simulink model "EcoSIM3_P2_C2_WIP"  (R2014b)
settings: Solver=ode1  SolverMode=SingleTasking  StartTime=0.0  StopTime=4  FixedStep=0.01  RelTol=1e-3
PostLoadFcn:
  | %, if any(exist('dsrtsu_mdlpostloadfcn', 'file') == [2, 3, 6]), try dsrtsu_mdlpostloadfcn('Execute', bdroot); catch fprintf('Error in PostLoadFcn (dsrtsu_mdlpostloadfcn) for model "%s":\n %s\n', bdroot, lasterr); end, end,
InitFcn:
  | tic
  | %Startup_EcoSIM
undefined symbols (not defined in the file or in its folder): canChannel, Controls, DriveCycles, Driver, EM_EFF_MAP, EM_PwrLoss_MAP, EngPwr, EngSpd, EngTrq, Glbl, Overwritten_Mode, Plants, Power, sigbuilder_block, Torque, Trialmap, Veh_Dynamics
libraries: simulink x135, canmsglib x113, fl_lib x104, canlib x89, nesl_utility x56, sdl_lib x29, dspsigops x6, dspswit3 x5, dspstat3 x2, commnoisgen2 x1, dspfdesign x1
(part 14 of 21)

== system EcoSIM3_P2_C2_WIP/Supervisory Controller/Supervisory_IO/VNT Kvaser/CAN Tx/ICE_BAS_Trans ==
  ICE_BAS_Trans : Inport
  Bus Selector1 : BusSelector  OutputSignals=ICE_Torque_Request_Nm,BAS_SoftECU_Receive.BAS_Mode_Request,BAS_SoftECU_Receive.BAS_Torque_Request_Nm,Trans_Receive.Gear_Request
  CAN Pack1 : canmsglib/CAN Pack  CANdbFile=C:\Users\EcoCAR_HIL\Documents\Khanna\EcoSIM3_P1_0_PHEV_TCU\Final_DBC\Engine_Transmission_BAS.dbc  MsgList=ECO_Engine_MSG101  MsgName=ECO_Engine_MSG101  MsgIDType=Standard (11-bit identifier)  MsgIdentifier=101  MsgLength=2  SignalInfo=ICE_Torque_Request_Nm$9$15$2$2$1$0$1.000000e-02$0$0$3.276700e+02$#  NSignals=1  StartBits=str2num('[int32(9)]')  SignalSizes=str2num('[int32(15)]')  ByteOrders=str2num('[int32(2)]')  DataTypes=str2num('[int32(2)]')  MultiplexTypes=str2num('[int32(1)]')  MultiplexValues=str2num('[double(0)]')  Factors=str2num('[double(1.000000e-02)]')  Offsets=str2num('[double(0)]')  Minimums=str2num('[double(0)]')  Maximums=str2num('[double(3.276700e+02)]')  Remote=off
      settings: DataFormat=CANdb specified signals
  CAN Pack2 : canmsglib/CAN Pack  CANdbFile=C:\Users\EcoCAR_HIL\Documents\Khanna\EcoSIM3_P1_0_PHEV_TCU\Final_DBC\Engine_Transmission_BAS.dbc  MsgList=ECO_BAS_Receive_MSG102  MsgName=ECO_BAS_Receive_MSG102  MsgIDType=Standard (11-bit identifier)  MsgIdentifier=102  MsgLength=2  SignalInfo=BAS_Mode_Request$8$1$2$2$1$0$1$0$0$1$#BAS_Torque_Request_Nm$9$15$2$1$1$0$1.000000e-02$0$-1.638400e+02$1.638300e+02$#  NSignals=2  StartBits=str2num('[int32(8);int32(9)]')  SignalSizes=str2num('[int32(1);int32(15)]')  ByteOrders=str2num('[int32(2);int32(2)]')  DataTypes=str2num('[int32(2);int32(1)]')  MultiplexTypes=str2num('[int32(1);int32(1)]')  MultiplexValues=str2num('[double(0);double(0)]')  Factors=str2num('[double(1);double(1.000000e-02)]')  Offsets=str2num('[double(0);double(0)]')  Minimums=str2num('[double(0);double(-1.638400e+02)]')  Maximums=str2num('[double(1);double(1.638300e+02)]')  Remote=off
      settings: DataFormat=CANdb specified signals
  CAN Pack3 : canmsglib/CAN Pack  CANdbFile=C:\Users\EcoCAR_HIL\Documents\Khanna\EcoSIM3_P1_0_PHEV_TCU\Final_DBC\Engine_Transmission_BAS.dbc  MsgList=ECO_Trans_Receive_MSG105  MsgName=ECO_Trans_Receive_MSG105  MsgIDType=Standard (11-bit identifier)  MsgIdentifier=105  MsgLength=1  SignalInfo=Clutch_Request$4$1$2$2$1$0$1$0$0$1$#Gear_Request$5$3$2$2$1$0$1$0$0$7$#  NSignals=2  StartBits=str2num('[int32(4);int32(5)]')  SignalSizes=str2num('[int32(1);int32(3)]')  ByteOrders=str2num('[int32(2);int32(2)]')  DataTypes=str2num('[int32(2);int32(2)]')  MultiplexTypes=str2num('[int32(1);int32(1)]')  MultiplexValues=str2num('[double(0);double(0)]')  Factors=str2num('[double(1);double(1)]')  Offsets=str2num('[double(0);double(0)]')  Minimums=str2num('[double(0);double(0)]')  Maximums=str2num('[double(1);double(7)]')  Remote=off
      settings: DataFormat=CANdb specified signals
  CAN Transmit1 : canlib/CAN Transmit  BlockHandle=7844.0023  DeviceMenu=Kvaser Virtual 1 (Channel 1)  Device=Kvaser Virtual 1 (Channel 1)  ObjConstructor=canChannel('Kvaser', 'Virtual 1', 1)  EnablePeriodicTransmit=off  MessagePeriod=1.000
  CAN Transmit2 : canlib/CAN Transmit  BlockHandle=7845.0023  DeviceMenu=Kvaser Virtual 1 (Channel 1)  Device=Kvaser Virtual 1 (Channel 1)  ObjConstructor=canChannel('Kvaser', 'Virtual 1', 1)  EnablePeriodicTransmit=off  MessagePeriod=1.000
  CAN Transmit3 : canlib/CAN Transmit  BlockHandle=7846.0023  DeviceMenu=Kvaser Virtual 1 (Channel 1)  Device=Kvaser Virtual 1 (Channel 1)  ObjConstructor=canChannel('Kvaser', 'Virtual 1', 1)  EnablePeriodicTransmit=off  MessagePeriod=1.000
  Ground1 : Ground
  Rate Transition{,1..3} (4 alike) : RateTransition
  wires:
  ICE_BAS_Trans/1 -> Bus Selector1/1
  Ground1/1 -> CAN Pack3/1
  CAN Pack2/1 -> CAN Transmit2/1
  Bus Selector1/3 -> Rate Transition2/1  "<BAS_Torque_Request_Nm>"
  Bus Selector1/2 -> Rate Transition1/1  "<BAS_Mode_Request>"
  CAN Pack3/1 -> CAN Transmit3/1
  Bus Selector1/4 -> Rate Transition3/1  "<Gear_Request>"
  CAN Pack1/1 -> CAN Transmit1/1
  Bus Selector1/1 -> Rate Transition/1  "<ICE_Torque_Request_Nm>"
  Rate Transition/1 -> CAN Pack1/1
  Rate Transition1/1 -> CAN Pack2/1
  Rate Transition2/1 -> CAN Pack2/2
  Rate Transition3/1 -> CAN Pack3/2

== system EcoSIM3_P2_C2_WIP/Supervisory Controller/Supervisory_IO/VNT Kvaser/CAN Tx/Mode ==
  Mode : Inport
  Bus Selector3 : BusSelector  OutputSignals=Supervisory.Mode
  CAN Pack5 : canmsglib/CAN Pack  CANdbFile=C:\Users\EcoCAR_HIL\Documents\Khanna\EcoSIM3_P1_0_PHEV_TCU\Final_DBC\EcoCAR3_Controls_Development.dbc  MsgList=MABx_Transmit_MSG094  MsgName=MABx_Transmit_MSG094  MsgIDType=Standard (11-bit identifier)  MsgIdentifier=94  MsgLength=1  SignalInfo=Mode$7$1$2$2$1$0$1$0$0$1$#  NSignals=1  StartBits=str2num('[int32(7)]')  SignalSizes=str2num('[int32(1)]')  ByteOrders=str2num('[int32(2)]')  DataTypes=str2num('[int32(2)]')  MultiplexTypes=str2num('[int32(1)]')  MultiplexValues=str2num('[double(0)]')  Factors=str2num('[double(1)]')  Offsets=str2num('[double(0)]')  Minimums=str2num('[double(0)]')  Maximums=str2num('[double(1)]')  Remote=off
      settings: DataFormat=CANdb specified signals
  CAN Transmit5 : canlib/CAN Transmit  BlockHandle=7869.0023  DeviceMenu=Kvaser Virtual 1 (Channel 1)  Device=Kvaser Virtual 1 (Channel 1)  ObjConstructor=canChannel('Kvaser', 'Virtual 1', 1)  EnablePeriodicTransmit=off  MessagePeriod=1.000
  Data Type Conversion1 : DataTypeConversion
  Rate Transition : RateTransition
  wires:
  Mode/1 -> Bus Selector3/1
  Data Type Conversion1/1 -> Rate Transition/1  "Mode"
  CAN Pack5/1 -> CAN Transmit5/1
  Bus Selector3/1 -> Data Type Conversion1/1  "<Mode>"
  Rate Transition/1 -> CAN Pack5/1

== system EcoSIM3_P2_C2_WIP/Supervisory Controller/Supervisory_IO/VNT Vector/CAN Rx/BAS ==
  Bus Creator : BusCreator  Inputs=2
  Bus Creator1 : BusCreator  Inputs=2
  Bus Creator2 : BusCreator  Inputs=3
  CAN Receive5 : canlib/CAN Receive  BlockHandle=17800.0002  DeviceMenu=Vector Virtual 1 (Channel 1)  Device=Vector Virtual 1 (Channel 1)  ObjConstructor=canChannel('Vector', 'Virtual 1', 1)  EnableStandardIDsFilter=off  StandardIDs=[257 273]  EnableExtendedIDsFilter=off  ExtendedIDs=0  SampleTime=0.01  MsgsPerTimestep=1  StdIDsCombo=Allow only  ExtIDsCombo=Block all  InternalFilterUpdateStatus=on
  CAN Unpack1 : canmsglib/CAN Unpack  CANdbFile=C:\Box Sync\EcoCAR 3\SMS\EcoSIM3_P2_C2\MIL\Final_DBC\InfineonInverter.dbc  MsgList=Status_1  MsgName=Status_1  MsgIDType=Standard (11-bit identifier)  MsgIdentifier=257  MsgLength=8  SignalInfo=Checksum3$0$8$1$2$1$0$1$0$-Inf$Inf$#CoolingReq$55$1$1$2$1$0$1$0$0$1$#Counter3$8$8$1$2$1$0$1$0$0$15$#ErrorInfo$48$2$1$2$1$0$1$0$0$3$#PowerRed$50$4$1$2$1$0$1$0$0$15$#ReadyHV$54$1$1$2$1$0$1$0$0$1$#RegAtLimit$56$1$1$2$1$0$1$0$0$1$#Reserved4$59$1$1$2$1$0$1$0$0$1$#SetLimitsOk$57$1$1$2$1$0$1$0$0$1$#SetValuesOk$58$1$1$2$1$0$1$0$0$1$#Speed$32$16$1$1$1$0$5.000000e-01$0$-16384$1.638350e+04$#StatusMode$60$4$1$2$1$0$1$0$0$15$#Torque_Normalized$16$16$1$1$1$0$3.051758e-05$0$-1$9.999695e-01$#  NSignals=13  IDPort=off  TimestampPort=off  ErrorPort=off  RemotePort=off  LengthPort=off  StatusPort=off  StartBits=str2num('[int32(0);int32(55);int32(8);int32(48);int32(50);int32(54);int32(56);int32(59);int32(57);int32(58);int32(32);int32(60);int32(16)]')  SignalSizes=str2num('[int32(8);int32(1);int32(8);int32(2);int32(4);int32(1);int32(1);int32(1);int32(1);int32(1);int32(16);int32(4);int32(16)]')  ByteOrders=str2num('[int32(1);int32(1);int32(1);int32(1);int32(1);int32(1);int32(1);int32(1);int32(1);int32(1);int32(1);int32(1);int32(1)]')  DataTypes=str2num('[int32(2);int32(2);int32(2);int32(2);int32(2);int32(2);int32(2);int32(2);int32(2);int32(2);int32(1);int32(2);int32(1)]')  MultiplexTypes=str2num('[int32(1);int32(1);int32(1);int32(1);int32(1);int32(1);int32(1);int32(1);int32(1);int32(1);int32(1);int32(1);int32(1)]')  MultiplexValues=str2num('[double(0);double(0);double(0);double(0);double(0);double(0);double(0);double(0);double(0);double(0);double(0);double(0);double(0)]')  Factors=str2num('[double(1);double(1);double(1);double(1);double(1);double(1);double(1);double(1);double(1);double(1);double(5.000000e-01);double(1);double(3.051758e-05)]')  Offsets=str2num('[double(0);double(0);double(0);double(0);double(0);double(0);double(0);double(0);double(0);double(0);double(0);double(0);double(0)]')  Minimums=str2num('[double(-Inf);double(0);double(0);double(0);double(0);double(0);double(0);double(0);double(0);double(0);double(-16384);double(0);double(-1)]')  Maximums=str2num('[double(Inf);double(1);double(15);double(3);double(15);double(1);double(1);double(1);double(1);double(1);double(1.638350e+04);double(15);double(9.999695e-01)]')
      settings: DataFormat=CANdb specified signals
  CAN Unpack2 : canmsglib/CAN Unpack  CANdbFile=C:\Box Sync\EcoCAR 3\SMS\EcoSIM3_P2_C2\MIL\Final_DBC\InfineonInverter.dbc  MsgList=Status_2  MsgName=Status_2  MsgIDType=Standard (11-bit identifier)  MsgIdentifier=273  MsgLength=8  SignalInfo=Checksum4$0$8$1$2$1$0$1$0$-Inf$Inf$#Counter4$8$4$1$2$1$0$1$0$0$15$#CurrentD_Limit$32$16$1$1$3$7$3.125000e-02$0$-1024$1.023969e+03$#CurrentD_Reference$32$16$1$1$3$9$3.125000e-02$0$-1024$1.023969e+03$#CurrentQ_Limit$32$16$1$1$3$6$3.125000e-02$0$-1024$1.023969e+03$#CurrentQ_Reference$32$16$1$1$3$8$3.125000e-02$0$-1024$1.023969e+03$#FaultU$13$1$1$2$1$0$1$0$0$1$#FaultV$14$1$1$2$1$0$1$0$0$1$#FaultW$15$1$1$2$1$0$1$0$0$1$#MultiplexCode$48$16$1$2$2$0$1$0$0$65535$#PhaseU_IGBT_Temp$32$16$1$1$3$3$7.812500e-03$0$-256$2.559922e+02$#PhaseV_IGBT_Temp$32$16$1$1$3$4$7.812500e-03$0$-256$2.559922e+02$#PhaseW_IGBT_Temp$32$16$1$1$3$5$7.812500e-03$0$-256$2.559922e+02$#RehabilitationReq$12$1$1$2$1$0$1$0$0$1$#Software_Version$32$16$1$2$3$0$1$0$0$65535$#Speed_Command$32$16$1$1$3$1$5.000000e-01$0$-16384$1.638350e+04$#Stator_Temperature$32$16$1$1$3$2$7.812500e-03$0$-256$2.559922e+02$#VoltageDC$16$16$1$1$1$0$3.125000e-02$0$-1024$1.023969e+03$#  NSignals=18  IDPort=off  TimestampPort=off  ErrorPort=off  RemotePort=off  LengthPort=off  StatusPort=off  StartBits=str2num('[int32(0);int32(8);int32(32);int32(32);int32(32);int32(32);int32(13);int32(14);int32(15);int32(48);int32(32);int32(32);int32(32);int32(12);int32(32);int32(32);int32(32);int32(16)]')  SignalSizes=str2num('[int32(8);int32(4);int32(16);int32(16);int32(16);int32(16);int32(1);int32(1);int32(1);int32(16);int32(16);int32(16);int32(16);int32(1);int32(16);int32(16);int32(16);int32(16)]')  ByteOrders=str2num('[int32(1);int32(1);int32(1);int32(1);int32(1);int32(1);int32(1);int32(1);int32(1);int32(1);int32(1);int32(1);int32(1);int32(1);int32(1);int32(1);int32(1);int32(1)]')  DataTypes=str2num('[int32(2);int32(2);int32(1);int32(1);int32(1);int32(1);int32(2);int32(2);int32(2);int32(2);int32(1);int32(1);int32(1);int32(2);int32(2);int32(1);int32(1);int32(1)]')  MultiplexTypes=str2num('[int32(1);int32(1);int32(3);int32(3);int32(3);int32(3);int32(1);int32(1);int32(1);int32(2);int32(3);int32(3);int32(3);int32(1);int32(3);int32(3);int32(3);int32(1)]')  MultiplexValues=str2num('[double(0);double(0);double(7);double(9);double(6);double(8);double(0);double(0);double(0);double(0);double(3);double(4);double(5);double(0);double(0);double(1);double(2);double(0)]')  Factors=str2num('[double(1);double(1);double(3.125000e-02);double(3.125000e-02);double(3.125000e-02);double(3.125000e-02);double(1);double(1);double(1);double(1);double(7.812500e-03);double(7.812500e-03);double(7.812500e-03);double(1);double(1);double(5.000000e-01);double(7.812500e-03);double(3.125000e-02)]')  Offsets=str2num('[double(0);double(0);double(0);double(0);double(0);double(0);double(0);double(0);double(0);double(0);double(0);double(0);double(0);double(0);double(0);double(0);double(0);double(0)]')  Minimums=str2num('[double(-Inf);double(0);double(-1024);double(-1024);double(-1024);double(-1024);double(0);double(0);double(0);double(0);double(-256);double(-256);double(-256);double(0);double(0);double(-16384);double(-256);double(-1024)]')  Maximums=str2num('[double(Inf);double(15);double(1.023969e+03);double(1.023969e+03);double(1.023969e+03);double(1.023969e+03);double(1);double(1);double(1);double(65535);double(2.559922e+02);double(2.559922e+02);double(2.559922e+02);double(1);double(65535);double(1.638350e+04);double(2.559922e+02);double(1.023969e+03)]')
      settings: DataFormat=CANdb specified signals
  Terminator2 : Terminator
  Terminator_{2..27} (26 alike) : Terminator
  BAS : Outport
  wires:
  CAN Unpack2/9 -> Bus Creator2/3  "Fault_W"
  CAN Unpack2/8 -> Bus Creator2/2  "Fault_V"
  CAN Unpack2/7 -> Bus Creator2/1  "Fault_U"
  CAN Unpack1/13 -> Bus Creator1/2  "BAS_Torque_Out_Nm"
  CAN Unpack1/11 -> Bus Creator1/1  "BAS_Speed_rad_per_s"
  Bus Creator1/1 -> Bus Creator/1  "Status_1"
  Bus Creator2/1 -> Bus Creator/2  "Status_2"
  Bus Creator/1 -> BAS/1  "BAS_CAN_Out"
  CAN Receive5/2 -> CAN Unpack1/1, CAN Unpack2/1
  CAN Receive5/1 -> Terminator2/1
  CAN Unpack1/1 -> Terminator_2/1
  CAN Unpack1/2 -> Terminator_3/1
  CAN Unpack1/3 -> Terminator_4/1
  CAN Unpack1/4 -> Terminator_5/1
  CAN Unpack1/5 -> Terminator_6/1
  CAN Unpack1/6 -> Terminator_7/1
  CAN Unpack1/7 -> Terminator_8/1
  CAN Unpack1/8 -> Terminator_9/1
  CAN Unpack1/9 -> Terminator_10/1
  CAN Unpack1/10 -> Terminator_11/1
  CAN Unpack1/12 -> Terminator_12/1
  CAN Unpack2/1 -> Terminator_13/1
  CAN Unpack2/2 -> Terminator_14/1
  CAN Unpack2/3 -> Terminator_15/1
  CAN Unpack2/4 -> Terminator_16/1
  CAN Unpack2/5 -> Terminator_17/1
  CAN Unpack2/6 -> Terminator_18/1
  CAN Unpack2/10 -> Terminator_19/1
  CAN Unpack2/11 -> Terminator_20/1
  CAN Unpack2/12 -> Terminator_21/1
  CAN Unpack2/13 -> Terminator_22/1
  CAN Unpack2/14 -> Terminator_23/1
  CAN Unpack2/15 -> Terminator_24/1
  CAN Unpack2/16 -> Terminator_25/1
  CAN Unpack2/17 -> Terminator_26/1
  CAN Unpack2/18 -> Terminator_27/1

== system EcoSIM3_P2_C2_WIP/Supervisory Controller/Supervisory_IO/VNT Vector/CAN Rx/Clutch Transmission ==
  Bus Creator : BusCreator  Inputs=1
  Bus Creator1 : BusCreator  Inputs=1
  Bus Creator2 : BusCreator  Inputs=2
  Bus Creator3 : BusCreator  Inputs=1
  CAN Receive3 : canlib/CAN Receive  BlockHandle=17875.0005  DeviceMenu=Vector Virtual 1 (Channel 1)  Device=Vector Virtual 1 (Channel 1)  ObjConstructor=canChannel('Vector', 'Virtual 1', 1)  EnableStandardIDsFilter=off  StandardIDs=[106 127]  EnableExtendedIDsFilter=off  ExtendedIDs=0  SampleTime=0.01  MsgsPerTimestep=all  StdIDsCombo=Allow only  ExtIDsCombo=Block all  InternalFilterUpdateStatus=on
  CAN Unpack1 : canmsglib/CAN Unpack  CANdbFile=C:\Box Sync\EcoCAR 3\SMS\EcoSIM3_P2_C2\MIL\Final_DBC\FTE_ElecHydAct.dbc  MsgList=CCU_HYB_01  MsgName=CCU_HYB_01  MsgIDType=Standard (11-bit identifier)  MsgIdentifier=127  MsgLength=8  SignalInfo=CY01_AngSpdCurr$24$9$1$2$1$0$200$-51000$-51000$50800$#CY01_Checksum$0$8$1$2$1$0$1$0$-Inf$Inf$#CY01_Counter$8$4$1$2$1$0$1$0$0$15$#CY01_ErrCAN$35$1$1$2$1$0$1$0$-Inf$Inf$#CY01_ErrHW$33$1$1$2$1$0$1$0$-Inf$Inf$#CY01_ErrMech$34$1$1$2$1$0$1$0$-Inf$Inf$#CY01_ErrTempHigh$38$1$1$2$1$0$1$0$-Inf$Inf$#CY01_ErrTempWarn$37$1$1$2$1$0$1$0$-Inf$Inf$#CY01_ErrUBattLow$36$1$1$2$1$0$1$0$-Inf$Inf$#CY01_SleepInd$39$1$1$2$1$0$1$0$-Inf$Inf$#CY01_i2trqCurr$12$12$1$2$1$0$2.500000e-01$-511$-511$5.122500e+02$#CY01_pCurr$56$8$1$2$1$0$2.000000e-01$0$0$5.060000e+01$#CY01_posCurr$40$13$1$2$1$0$1$0$0$8191$#CY01_stMode$53$3$1$2$1$0$1$0$0$7$#  NSignals=14  IDPort=off  TimestampPort=off  ErrorPort=off  RemotePort=off  LengthPort=off  StatusPort=off  StartBits=str2num('[int32(24);int32(0);int32(8);int32(35);int32(33);int32(34);int32(38);int32(37);int32(36);int32(39);int32(12);int32(56);int32(40);int32(53)]')  SignalSizes=str2num('[int32(9);int32(8);int32(4);int32(1);int32(1);int32(1);int32(1);int32(1);int32(1);int32(1);int32(12);int32(8);int32(13);int32(3)]')  ByteOrders=str2num('[int32(1);int32(1);int32(1);int32(1);int32(1);int32(1);int32(1);int32(1);int32(1);int32(1);int32(1);int32(1);int32(1);int32(1)]')  DataTypes=str2num('[int32(2);int32(2);int32(2);int32(2);int32(2);int32(2);int32(2);int32(2);int32(2);int32(2);int32(2);int32(2);int32(2);int32(2)]')  MultiplexTypes=str2num('[int32(1);int32(1);int32(1);int32(1);int32(1);int32(1);int32(1);int32(1);int32(1);int32(1);int32(1);int32(1);int32(1);int32(1)]')  MultiplexValues=str2num('[double(0);double(0);double(0);double(0);double(0);double(0);double(0);double(0);double(0);double(0);double(0);double(0);double(0);double(0)]')  Factors=str2num('[double(200);double(1);double(1);double(1);double(1);double(1);double(1);double(1);double(1);double(1);double(2.500000e-01);double(2.000000e-01);double(1);double(1)]')  Offsets=str2num('[double(-51000);double(0);double(0);double(0);double(0);double(0);double(0);double(0);double(0);double(0);double(-511);double(0);double(0);double(0)]')  Minimums=str2num('[double(-51000);double(-Inf);double(0);double(-Inf);double(-Inf);double(-Inf);double(-Inf);double(-Inf);double(-Inf);double(-Inf);double(-511);double(0);double(0);double(0)]')  Maximums=str2num('[double(50800);double(Inf);double(15);double(Inf);double(Inf);double(Inf);double(Inf);double(Inf);double(Inf);double(Inf);double(5.122500e+02);double(5.060000e+01);double(8191);double(7)]')
      settings: DataFormat=CANdb specified signals
  CAN Unpack3 : canmsglib/CAN Unpack  CANdbFile=C:\Users\EcoCAR_HIL\Documents\Khanna\EcoSIM3_P1_0_PHEV_TCU\Final_DBC\Engine_Transmission_BAS.dbc  MsgList=ECO_Trans_Status_MSG106  MsgName=ECO_Trans_Status_MSG106  MsgIDType=Standard (11-bit identifier)  MsgIdentifier=106  MsgLength=1  SignalInfo=Actual_Gear$1$3$2$2$1$0$1$0$0$7$#Clutch_Sw$7$1$2$2$1$0$1$0$0$1$#TCM_Gear$4$3$2$2$1$0$1$0$0$7$#  NSignals=3  IDPort=off  TimestampPort=off  ErrorPort=off  RemotePort=off  LengthPort=off  StatusPort=off  StartBits=str2num('[int32(1);int32(7);int32(4)]')  SignalSizes=str2num('[int32(3);int32(1);int32(3)]')  ByteOrders=str2num('[int32(2);int32(2);int32(2)]')  DataTypes=str2num('[int32(2);int32(2);int32(2)]')  MultiplexTypes=str2num('[int32(1);int32(1);int32(1)]')  MultiplexValues=str2num('[double(0);double(0);double(0)]')  Factors=str2num('[double(1);double(1);double(1)]')  Offsets=str2num('[double(0);double(0);double(0)]')  Minimums=str2num('[double(0);double(0);double(0)]')  Maximums=str2num('[double(7);double(1);double(7)]')
      settings: DataFormat=CANdb specified signals
  Scope : Scope
      settings: SaveName=ScopeData49
  Scope1 : Scope
      settings: SaveName=ScopeData50
  Terminator12 : Terminator
  Terminator28 : Terminator
  Terminator29 : Terminator
  Trans : Outport
  CP1 : Outport  Port=2
  wires:
  CAN Receive3/1 -> Terminator12/1
  CAN Unpack3/1 -> Bus Creator1/1  "Actual_Gear"
  CAN Receive3/2 -> CAN Unpack1/1, CAN Unpack3/1
  CAN Unpack3/2 -> Terminator28/1  "Clutch_Sw"
  CAN Unpack3/3 -> Terminator29/1  "TCM_Gear"
  Bus Creator1/1 -> Bus Creator/1  "Message_1"
  Bus Creator/1 -> Trans/1  "Clutch_Transmission_CAN_Out"
  CAN Unpack1/13 -> Scope/1, Bus Creator2/1  "CY01_posCurr"
  CAN Unpack1/14 -> Scope1/1, Bus Creator2/2  "CY01_stMode"
  Bus Creator2/1 -> Bus Creator3/1  "CCU_HYB_01"
  Bus Creator3/1 -> CP1/1  "CP1_CAN_Out"

== system EcoSIM3_P2_C2_WIP/Supervisory Controller/Supervisory_IO/VNT Vector/CAN Rx/ESS ==
  Bus Creator : BusCreator  Inputs=3
  Bus Creator1 : BusCreator  Inputs=12
  Bus Creator2 : BusCreator
  Bus Creator3 : BusCreator  Inputs=2
  Bus Creator4 : BusCreator  Inputs=1
  CAN Receive1 : canlib/CAN Receive  BlockHandle=17908.0005  DeviceMenu=Kvaser Virtual 1 (Channel 1)  Device=Vector Virtual 1 (Channel 1)  ObjConstructor=canChannel('Vector', 'Virtual 1', 1)  EnableStandardIDsFilter=off  StandardIDs=1072  EnableExtendedIDsFilter=off  ExtendedIDs=0  SampleTime=0.01  MsgsPerTimestep=1  StdIDsCombo=Allow only  ExtIDsCombo=Block all  InternalFilterUpdateStatus=on
  CAN Receive2 : canlib/CAN Receive  BlockHandle=17909.0001  DeviceMenu=Kvaser Virtual 1 (Channel 1)  Device=Vector Virtual 1 (Channel 1)  ObjConstructor=canChannel('Vector', 'Virtual 1', 1)  EnableStandardIDsFilter=off  StandardIDs=1040  EnableExtendedIDsFilter=off  ExtendedIDs=0  SampleTime=0.01  MsgsPerTimestep=1  StdIDsCombo=Allow only  ExtIDsCombo=Block all  InternalFilterUpdateStatus=on
  CAN Receive3 : canlib/CAN Receive  BlockHandle=17910.0001  DeviceMenu=Kvaser Virtual 1 (Channel 1)  Device=Vector Virtual 1 (Channel 1)  ObjConstructor=canChannel('Vector', 'Virtual 1', 1)  EnableStandardIDsFilter=off  StandardIDs=1056  EnableExtendedIDsFilter=off  ExtendedIDs=0  SampleTime=0.01  MsgsPerTimestep=1  StdIDsCombo=Allow only  ExtIDsCombo=Block all  InternalFilterUpdateStatus=on
  CAN Receive4 : canlib/CAN Receive  BlockHandle=17911.0001  DeviceMenu=Kvaser Virtual 1 (Channel 1)  Device=Vector Virtual 1 (Channel 1)  ObjConstructor=canChannel('Vector', 'Virtual 1', 1)  EnableStandardIDsFilter=off  StandardIDs=1088  EnableExtendedIDsFilter=off  ExtendedIDs=0  SampleTime=0.01  MsgsPerTimestep=1  StdIDsCombo=Allow only  ExtIDsCombo=Block all  InternalFilterUpdateStatus=on
  CAN Unpack1 : canmsglib/CAN Unpack  CANdbFile=C:\Users\EcoCAR_HIL\Documents\Khanna\EcoSIM3_P1_0_PHEV_TCU\Final_DBC\BCM_VehBus_Std.dbc  MsgList=BCM_Limits  MsgName=BCM_Limits  MsgIDType=Standard (11-bit identifier)  MsgIdentifier=1056  MsgLength=8  SignalInfo=bcm_cell_overvolt$55$1$2$2$1$0$1$0$0$1$#bcm_cell_undervolt$54$1$2$2$1$0$1$0$0$1$#bcm_chg_buf$32$8$2$2$1$0$5.000000e-01$0$0$100$#bcm_chg_max$16$12$2$2$1$0$2.500000e-01$0$0$1000$#bcm_dis_buf$24$8$2$2$1$0$5.000000e-01$0$0$100$#bcm_dis_max$12$12$2$2$1$0$2.500000e-01$0$0$1000$#bcm_t_coolant$40$8$2$2$1$0$5.000000e-01$-40$-40$85$#  NSignals=7  IDPort=off  TimestampPort=off  ErrorPort=off  RemotePort=off  LengthPort=off  StatusPort=off  StartBits=str2num('[int32(55);int32(54);int32(32);int32(16);int32(24);int32(12);int32(40)]')  SignalSizes=str2num('[int32(1);int32(1);int32(8);int32(12);int32(8);int32(12);int32(8)]')  ByteOrders=str2num('[int32(2);int32(2);int32(2);int32(2);int32(2);int32(2);int32(2)]')  DataTypes=str2num('[int32(2);int32(2);int32(2);int32(2);int32(2);int32(2);int32(2)]')  MultiplexTypes=str2num('[int32(1);int32(1);int32(1);int32(1);int32(1);int32(1);int32(1)]')  MultiplexValues=str2num('[double(0);double(0);double(0);double(0);double(0);double(0);double(0)]')  Factors=str2num('[double(1);double(1);double(5.000000e-01);double(2.500000e-01);double(5.000000e-01);double(2.500000e-01);double(5.000000e-01)]')  Offsets=str2num('[double(0);double(0);double(0);double(0);double(0);double(0);double(-40)]')  Minimums=str2num('[double(0);double(0);double(0);double(0);double(0);double(0);double(-40)]')  Maximums=str2num('[double(1);double(1);double(100);double(1000);double(100);double(1000);double(85)]')
      settings: DataFormat=CANdb specified signals
  CAN Unpack2 : canmsglib/CAN Unpack  CANdbFile=C:\Users\EcoCAR_HIL\Documents\Khanna\EcoSIM3_P1_0_PHEV_TCU\Final_DBC\BCM_VehBus_Std.dbc  MsgList=BCM_Status  MsgName=BCM_Status  MsgIDType=Standard (11-bit identifier)  MsgIdentifier=1040  MsgLength=8  SignalInfo=bcm_alarm$14$2$2$2$1$0$1$0$0$3$#bcm_chg_done$52$1$2$2$1$0$1$0$0$1$#bcm_chgc_stat$6$2$2$2$1$0$1$0$0$2$#bcm_cool_req$53$1$2$2$1$0$1$0$0$1$#bcm_cpwr_cmd$12$1$2$2$1$0$1$0$0$1$#bcm_cpwr_mon$13$1$2$2$1$0$1$0$0$1$#bcm_epo$1$1$2$2$1$0$1$0$0$1$#bcm_gfd$16$12$2$2$1$0$2.500000e-01$0$0$1000$#bcm_hvil_mon$3$1$2$2$1$0$1$0$0$1$#bcm_ibat$40$16$2$2$1$0$2.500000e-02$-1000$-1000$500$#bcm_lls_status$54$2$2$2$1$0$1$0$0$3$#bcm_mainc_stat$4$2$2$2$1$0$1$0$0$2$#bcm_on_plug$2$1$2$2$1$0$1$0$0$1$#bcm_ready$0$1$2$2$1$0$1$0$0$1$#bcm_soc$24$8$2$2$1$0$5.000000e-01$0$0$100$#bcm_vbat$56$12$2$2$1$0$2.500000e-01$0$0$1000$#  NSignals=16  IDPort=off  TimestampPort=off  ErrorPort=off  RemotePort=off  LengthPort=off  StatusPort=off  StartBits=str2num('[int32(14);int32(52);int32(6);int32(53);int32(12);int32(13);int32(1);int32(16);int32(3);int32(40);int32(54);int32(4);int32(2);int32(0);int32(24);int32(56)]')  SignalSizes=str2num('[int32(2);int32(1);int32(2);int32(1);int32(1);int32(1);int32(1);int32(12);int32(1);int32(16);int32(2);int32(2);int32(1);int32(1);int32(8);int32(12)]')  ByteOrders=str2num('[int32(2);int32(2);int32(2);int32(2);int32(2);int32(2);int32(2);int32(2);int32(2);int32(2);int32(2);int32(2);int32(2);int32(2);int32(2);int32(2)]')  DataTypes=str2num('[int32(2);int32(2);int32(2);int32(2);int32(2);int32(2);int32(2);int32(2);int32(2);int32(2);int32(2);int32(2);int32(2);int32(2);int32(2);int32(2)]')  MultiplexTypes=str2num('[int32(1);int32(1);int32(1);int32(1);int32(1);int32(1);int32(1);int32(1);int32(1);int32(1);int32(1);int32(1);int32(1);int32(1);int32(1);int32(1)]')  MultiplexValues=str2num('[double(0);double(0);double(0);double(0);double(0);double(0);double(0);double(0);double(0);double(0);double(0);double(0);double(0);double(0);double(0);double(0)]')  Factors=str2num('[double(1);double(1);double(1);double(1);double(1);double(1);double(1);double(2.500000e-01);double(1);double(2.500000e-02);double(1);double(1);double(1);double(1);double(5.000000e-01);double(2.500000e-01)]')  Offsets=str2num('[double(0);double(0);double(0);double(0);double(0);double(0);double(0);double(0);double(0);double(-1000);double(0);double(0);double(0);double(0);double(0);double(0)]')  Minimums=str2num('[double(0);double(0);double(0);double(0);double(0);double(0);double(0);double(0);double(0);double(-1000);double(0);double(0);double(0);double(0);double(0);double(0)]')  Maximums=str2num('[double(3);double(1);double(2);double(1);double(1);double(1);double(1);double(1000);double(1);double(500);double(3);double(2);double(1);double(1);double(100);double(1000)]')
      settings: DataFormat=CANdb specified signals
  CAN Unpack3 : canmsglib/CAN Unpack  CANdbFile=C:\Users\EcoCAR_HIL\Documents\Khanna\EcoSIM3_P1_0_PHEV_TCU\Final_DBC\BCM_VehBus_Std.dbc  MsgList=BCM_Data2  MsgName=BCM_Data2  MsgIDType=Standard (11-bit identifier)  MsgIdentifier=1088  MsgLength=8  SignalInfo=bcm_balancing$7$1$2$2$1$0$1$0$0$1$#bcm_balancing_cnt$56$8$2$2$1$0$1$0$0$250$#bcm_eeprom_wip$0$1$2$2$1$0$1$0$0$1$#bcm_fault_mon$6$1$2$2$1$0$1$0$0$1$#bcm_fgd$8$8$2$2$1$0$5.000000e-01$0$0$100$#bcm_ibat2$24$16$2$2$1$0$2.500000e-02$-1000$-1000$500$#bcm_mainc_step$2$4$2$2$1$0$1$0$0$15$#bcm_vbus_neg$48$12$2$2$1$0$2.500000e-01$-500$-500$500$#bcm_vbus_pos$44$12$2$2$1$0$2.500000e-01$0$0$1000$#  NSignals=9  IDPort=off  TimestampPort=off  ErrorPort=off  RemotePort=off  LengthPort=off  StatusPort=off  StartBits=str2num('[int32(7);int32(56);int32(0);int32(6);int32(8);int32(24);int32(2);int32(48);int32(44)]')  SignalSizes=str2num('[int32(1);int32(8);int32(1);int32(1);int32(8);int32(16);int32(4);int32(12);int32(12)]')  ByteOrders=str2num('[int32(2);int32(2);int32(2);int32(2);int32(2);int32(2);int32(2);int32(2);int32(2)]')  DataTypes=str2num('[int32(2);int32(2);int32(2);int32(2);int32(2);int32(2);int32(2);int32(2);int32(2)]')  MultiplexTypes=str2num('[int32(1);int32(1);int32(1);int32(1);int32(1);int32(1);int32(1);int32(1);int32(1)]')  MultiplexValues=str2num('[double(0);double(0);double(0);double(0);double(0);double(0);double(0);double(0);double(0)]')  Factors=str2num('[double(1);double(1);double(1);double(1);double(5.000000e-01);double(2.500000e-02);double(1);double(2.500000e-01);double(2.500000e-01)]')  Offsets=str2num('[double(0);double(0);double(0);double(0);double(0);double(-1000);double(0);double(-500);double(0)]')  Minimums=str2num('[double(0);double(0);double(0);double(0);double(0);double(-1000);double(0);double(-500);double(0)]')  Maximums=str2num('[double(1);double(250);double(1);double(1);double(100);double(500);double(15);double(500);double(1000)]')
      settings: DataFormat=CANdb specified signals
  CAN Unpack6 : canmsglib/CAN Unpack  CANdbFile=C:\Users\EcoCAR_HIL\Documents\Khanna\EcoSIM3_P1_0_PHEV_TCU\Final_DBC\BCM_VehBus_Std.dbc  MsgList=BCM_Data1  MsgName=BCM_Data1  MsgIDType=Standard (11-bit identifier)  MsgIdentifier=1072  MsgLength=8  SignalInfo=bcm_cell_tmax$32$8$2$2$1$0$5.000000e-01$-40$-40$85$#bcm_cell_tmin$40$8$2$2$1$0$5.000000e-01$-40$-40$85$#bcm_cell_vmax$8$13$2$2$1$0$1.000000e-03$0$0$5$#bcm_cell_vmin$24$13$2$2$1$0$1.000000e-03$0$0$5$#bcm_chga_ena$7$1$2$2$1$0$1$0$0$1$#bcm_chga_mon$22$1$2$2$1$0$1$0$0$1$#bcm_lvbat$56$8$2$2$1$0$1.000000e-01$0$0$25$#bcm_mod_ena$23$1$2$2$1$0$1$0$0$1$#bcm_veh_mon$21$1$2$2$1$0$1$0$0$1$#  NSignals=9  IDPort=off  TimestampPort=off  ErrorPort=off  RemotePort=off  LengthPort=off  StatusPort=off  StartBits=str2num('[int32(32);int32(40);int32(8);int32(24);int32(7);int32(22);int32(56);int32(23);int32(21)]')  SignalSizes=str2num('[int32(8);int32(8);int32(13);int32(13);int32(1);int32(1);int32(8);int32(1);int32(1)]')  ByteOrders=str2num('[int32(2);int32(2);int32(2);int32(2);int32(2);int32(2);int32(2);int32(2);int32(2)]')  DataTypes=str2num('[int32(2);int32(2);int32(2);int32(2);int32(2);int32(2);int32(2);int32(2);int32(2)]')  MultiplexTypes=str2num('[int32(1);int32(1);int32(1);int32(1);int32(1);int32(1);int32(1);int32(1);int32(1)]')  MultiplexValues=str2num('[double(0);double(0);double(0);double(0);double(0);double(0);double(0);double(0);double(0)]')  Factors=str2num('[double(5.000000e-01);double(5.000000e-01);double(1.000000e-03);double(1.000000e-03);double(1);double(1);double(1.000000e-01);double(1);double(1)]')  Offsets=str2num('[double(-40);double(-40);double(0);double(0);double(0);double(0);double(0);double(0);double(0)]')  Minimums=str2num('[double(-40);double(-40);double(0);double(0);double(0);double(0);double(0);double(0);double(0)]')  Maximums=str2num('[double(85);double(85);double(5);double(5);double(1);double(1);double(25);double(1);double(1)]')
      settings: DataFormat=CANdb specified signals
  Terminator{1..3,5..9,33..38} (14 alike) : Terminator
  Terminator_{15..19} (5 alike) : Terminator
  ESSTransmit : Outport
  wires:
  CAN Receive2/1 -> Terminator2/1
  Bus Creator2/1 -> ESSTransmit/1  "ESS_CAN_Out"
  CAN Unpack2/1 -> Terminator3/1
  CAN Unpack2/2 -> Bus Creator1/1  "bcm_chg_done"
  CAN Unpack2/4 -> Terminator5/1
  CAN Unpack2/8 -> Terminator6/1
  CAN Unpack2/11 -> Terminator8/1
  CAN Unpack2/13 -> Bus Creator1/9  "bcm_on_plug"
  CAN Unpack6/1 -> Bus Creator/1  "bcm_cell_tmax"
  CAN Unpack6/2 -> Bus Creator/2  "bcm_cell_tmin"
  CAN Unpack6/3 -> Terminator33/1
  CAN Unpack6/4 -> Terminator34/1
  CAN Unpack6/5 -> Terminator35/1
  CAN Unpack6/6 -> Terminator36/1
  CAN Unpack6/7 -> Terminator37/1
  CAN Unpack6/8 -> Terminator38/1
  CAN Unpack6/9 -> Bus Creator/3  "bcm_veh_mon"
  CAN Unpack2/3 -> Bus Creator1/2  "bcm_chgc_stat"
  CAN Unpack2/5 -> Bus Creator1/3  "bcm_cpwr_cmd"
  CAN Unpack2/6 -> Bus Creator1/4  "bcm_cpwr_mon"
  CAN Unpack2/7 -> Bus Creator1/5  "bcm_epo"
  CAN Unpack2/9 -> Bus Creator1/6  "bcm_hvil_mon"
  CAN Unpack2/10 -> Bus Creator1/7  "bcm_ibat"
  CAN Unpack2/12 -> Bus Creator1/8  "bcm_mainc_stat"
  CAN Unpack2/14 -> Bus Creator1/10  "bcm_ready"
  CAN Unpack2/15 -> Bus Creator1/11  "bcm_soc"
  CAN Unpack2/16 -> Bus Creator1/12  "bcm_vbat"
  CAN Unpack1/3 -> Bus Creator3/1  "bcm_chg_buf"
  CAN Unpack1/5 -> Bus Creator3/2  "bcm_dis_buf"
  Bus Creator1/1 -> Bus Creator2/1  "BCM_Status"
  Bus Creator/1 -> Bus Creator2/2  "BCM_Data1"
  Bus Creator3/1 -> Bus Creator2/4  "BCM_Limits"
  CAN Unpack1/1 -> Terminator_15/1
  CAN Unpack1/2 -> Terminator_16/1
  CAN Unpack1/4 -> Terminator_17/1
  CAN Unpack1/6 -> Terminator_18/1
  CAN Unpack1/7 -> Terminator_19/1
  CAN Receive1/1 -> Terminator1/1
  CAN Receive3/1 -> Terminator7/1
  CAN Receive2/2 -> CAN Unpack2/1
  CAN Receive1/2 -> CAN Unpack6/1
  CAN Receive3/2 -> CAN Unpack1/1
  CAN Receive4/2 -> CAN Unpack3/1
  CAN Receive4/1 -> Terminator9/1
  CAN Unpack3/1 -> Bus Creator4/1  "bcm_balancing"
  Bus Creator4/1 -> Bus Creator2/3  "BCM_Data2"

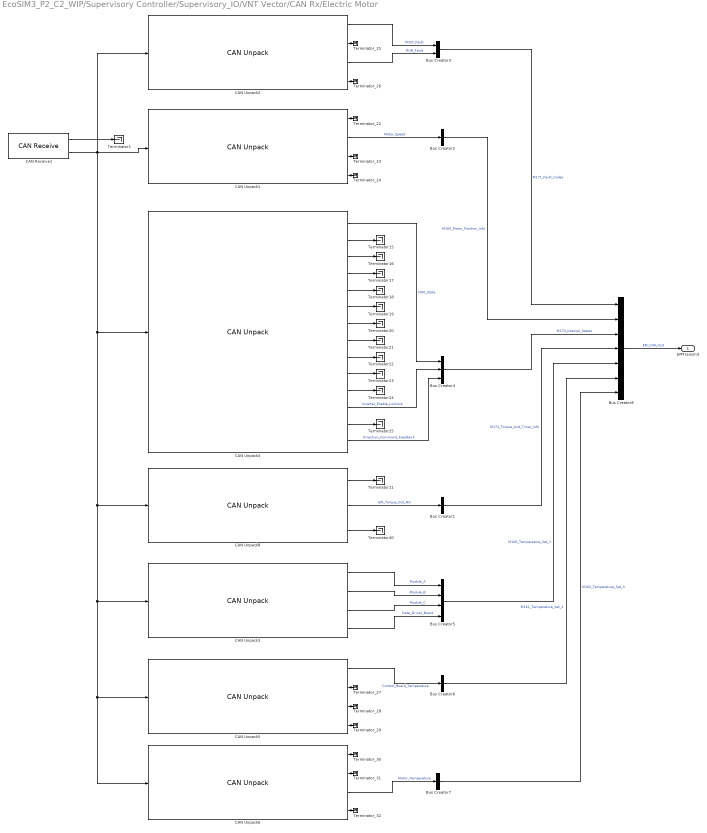
== system EcoSIM3_P2_C2_WIP/Supervisory Controller/Supervisory_IO/VNT Vector/CAN Rx/Electric Motor ==
  Bus Creator{1..2,6..7} (4 alike) : BusCreator  Inputs=1
  Bus Creator3 : BusCreator  Inputs=2
  Bus Creator4 : BusCreator  Inputs=3
  Bus Creator5 : BusCreator
  Bus Creator8 : BusCreator  Inputs=7
  CAN Receive1 : canlib/CAN Receive  BlockHandle=17991.0001  DeviceMenu=Vector Virtual 1 (Channel 2)  Device=Vector Virtual 1 (Channel 2)  ObjConstructor=canChannel('Vector', 'Virtual 1', 2)  EnableStandardIDsFilter=off  StandardIDs=[160 161 162 165 170 171 172]  EnableExtendedIDsFilter=off  ExtendedIDs=0  SampleTime=0.01  MsgsPerTimestep=1  StdIDsCombo=Allow only  ExtIDsCombo=Block all  InternalFilterUpdateStatus=on
  CAN Unpack1 : canmsglib/CAN Unpack  CANdbFile=C:\Users\EcoCAR_HIL\Documents\Khanna\EcoSIM3_P1_0_PHEV_TCU\Final_DBC\20160113 RMS PM CAN DB.dbc  MsgList=M165_Motor_Position_Info  MsgName=M165_Motor_Position_Info  MsgIDType=Standard (11-bit identifier)  MsgIdentifier=165  MsgLength=8  SignalInfo=D1_Motor_Angle_Electrical$0$16$1$2$1$0$1.000000e-01$0$0$6.553500e+03$#D2_Motor_Speed$16$16$1$1$1$0$1$0$-32768$32767$#D3_Electrical_Output_Frequency$32$16$1$1$1$0$1.000000e-01$0$-3.276800e+03$3.276700e+03$#D4_Delta_Resolver_Filtered$48$16$1$1$1$0$1.000000e-01$0$-3.276800e+03$3.276700e+03$#  NSignals=4  IDPort=off  TimestampPort=off  ErrorPort=off  RemotePort=off  LengthPort=off  StatusPort=off  StartBits=str2num('[int32(0);int32(16);int32(32);int32(48)]')  SignalSizes=str2num('[int32(16);int32(16);int32(16);int32(16)]')  ByteOrders=str2num('[int32(1);int32(1);int32(1);int32(1)]')  DataTypes=str2num('[int32(2);int32(1);int32(1);int32(1)]')  MultiplexTypes=str2num('[int32(1);int32(1);int32(1);int32(1)]')  MultiplexValues=str2num('[double(0);double(0);double(0);double(0)]')  Factors=str2num('[double(1.000000e-01);double(1);double(1.000000e-01);double(1.000000e-01)]')  Offsets=str2num('[double(0);double(0);double(0);double(0)]')  Minimums=str2num('[double(0);double(-32768);double(-3.276800e+03);double(-3.276800e+03)]')  Maximums=str2num('[double(6.553500e+03);double(32767);double(3.276700e+03);double(3.276700e+03)]')
      settings: DataFormat=CANdb specified signals
  CAN Unpack2 : canmsglib/CAN Unpack  CANdbFile=C:\Users\EcoCAR_HIL\Documents\Khanna\EcoSIM3_P1_0_PHEV_TCU\Final_DBC\20160113 RMS PM CAN DB.dbc  MsgList=M171_Fault_Codes  MsgName=M171_Fault_Codes  MsgIDType=Standard (11-bit identifier)  MsgIdentifier=171  MsgLength=8  SignalInfo=D1_Post_Fault_Lo$0$16$1$2$1$0$1$0$0$65535$#D2_Post_Fault_Hi$16$16$1$2$1$0$1$0$0$65535$#D3_Run_Fault_Lo$32$16$1$2$1$0$1$0$0$65535$#D4_Run_Fault_Hi$48$16$1$2$1$0$1$0$0$65535$#  NSignals=4  IDPort=off  TimestampPort=off  ErrorPort=off  RemotePort=off  LengthPort=off  StatusPort=off  StartBits=str2num('[int32(0);int32(16);int32(32);int32(48)]')  SignalSizes=str2num('[int32(16);int32(16);int32(16);int32(16)]')  ByteOrders=str2num('[int32(1);int32(1);int32(1);int32(1)]')  DataTypes=str2num('[int32(2);int32(2);int32(2);int32(2)]')  MultiplexTypes=str2num('[int32(1);int32(1);int32(1);int32(1)]')  MultiplexValues=str2num('[double(0);double(0);double(0);double(0)]')  Factors=str2num('[double(1);double(1);double(1);double(1)]')  Offsets=str2num('[double(0);double(0);double(0);double(0)]')  Minimums=str2num('[double(0);double(0);double(0);double(0)]')  Maximums=str2num('[double(65535);double(65535);double(65535);double(65535)]')
      settings: DataFormat=CANdb specified signals
  CAN Unpack3 : canmsglib/CAN Unpack  CANdbFile=C:\Users\EcoCAR_HIL\Documents\Khanna\EcoSIM3_P1_0_PHEV_TCU\Final_DBC\20160113 RMS PM CAN DB.dbc  MsgList=M160_Temperature_Set_1  MsgName=M160_Temperature_Set_1  MsgIDType=Standard (11-bit identifier)  MsgIdentifier=160  MsgLength=8  SignalInfo=D1_Module_A$0$16$1$1$1$0$1.000000e-01$0$-3.276800e+03$3.276700e+03$#D2_Module_B$16$16$1$1$1$0$1.000000e-01$0$-3.276800e+03$3.276700e+03$#D3_Module_C$32$16$1$1$1$0$1.000000e-01$0$-3.276800e+03$3.276700e+03$#D4_Gate_Driver_Board$48$16$1$1$1$0$1.000000e-01$0$-3.276800e+03$3.276700e+03$#  NSignals=4  IDPort=off  TimestampPort=off  ErrorPort=off  RemotePort=off  LengthPort=off  StatusPort=off  StartBits=str2num('[int32(0);int32(16);int32(32);int32(48)]')  SignalSizes=str2num('[int32(16);int32(16);int32(16);int32(16)]')  ByteOrders=str2num('[int32(1);int32(1);int32(1);int32(1)]')  DataTypes=str2num('[int32(1);int32(1);int32(1);int32(1)]')  MultiplexTypes=str2num('[int32(1);int32(1);int32(1);int32(1)]')  MultiplexValues=str2num('[double(0);double(0);double(0);double(0)]')  Factors=str2num('[double(1.000000e-01);double(1.000000e-01);double(1.000000e-01);double(1.000000e-01)]')  Offsets=str2num('[double(0);double(0);double(0);double(0)]')  Minimums=str2num('[double(-3.276800e+03);double(-3.276800e+03);double(-3.276800e+03);double(-3.276800e+03)]')  Maximums=str2num('[double(3.276700e+03);double(3.276700e+03);double(3.276700e+03);double(3.276700e+03)]')
      settings: DataFormat=CANdb specified signals
  CAN Unpack4 : canmsglib/CAN Unpack  CANdbFile=C:\Users\EcoCAR_HIL\Documents\Khanna\EcoSIM3_P1_0_PHEV_TCU\Final_DBC\20160113 RMS PM CAN DB.dbc  MsgList=M170_Internal_States  MsgName=M170_Internal_States  MsgIDType=Standard (11-bit identifier)  MsgIdentifier=170  MsgLength=8  SignalInfo=D1_VSM_State$0$16$1$2$1$0$1$0$0$15$#D2_Inverter_State$16$8$1$2$1$0$1$0$0$255$#D3_Relay_1_Status$24$1$1$2$1$0$1$0$0$1$#D3_Relay_2_Status$25$1$1$2$1$0$1$0$0$1$#D3_Relay_3_Status$26$1$1$2$1$0$1$0$0$1$#D3_Relay_4_Status$27$1$1$2$1$0$1$0$0$1$#D3_Relay_5_Status$28$1$1$2$1$0$1$0$-Inf$Inf$#D3_Relay_6_Status$29$1$1$2$1$0$1$0$-Inf$Inf$#D4_Inverter_Discharge_State$37$3$1$2$1$0$1$0$0$7$#D4_Inverter_Run_Mode$32$1$1$2$1$0$1$0$0$1$#D5_Inverter_Command_Mode$40$1$1$2$1$0$1$0$0$1$#D6_Inverter_Enable_Lockout$55$1$1$2$1$0$1$0$0$1$#D6_Inverter_Enable_State$48$1$1$2$1$0$1$0$0$1$#D7_Direction_Command$56$8$1$2$1$0$1$0$0$1$#  NSignals=14  IDPort=off  TimestampPort=off  ErrorPort=off  RemotePort=off  LengthPort=off  StatusPort=off  StartBits=str2num('[int32(0);int32(16);int32(24);int32(25);int32(26);int32(27);int32(28);int32(29);int32(37);int32(32);int32(40);int32(55);int32(48);int32(56)]')  SignalSizes=str2num('[int32(16);int32(8);int32(1);int32(1);int32(1);int32(1);int32(1);int32(1);int32(3);int32(1);int32(1);int32(1);int32(1);int32(8)]')  ByteOrders=str2num('[int32(1);int32(1);int32(1);int32(1);int32(1);int32(1);int32(1);int32(1);int32(1);int32(1);int32(1);int32(1);int32(1);int32(1)]')  DataTypes=str2num('[int32(2);int32(2);int32(2);int32(2);int32(2);int32(2);int32(2);int32(2);int32(2);int32(2);int32(2);int32(2);int32(2);int32(2)]')  MultiplexTypes=str2num('[int32(1);int32(1);int32(1);int32(1);int32(1);int32(1);int32(1);int32(1);int32(1);int32(1);int32(1);int32(1);int32(1);int32(1)]')  MultiplexValues=str2num('[double(0);double(0);double(0);double(0);double(0);double(0);double(0);double(0);double(0);double(0);double(0);double(0);double(0);double(0)]')  Factors=str2num('[double(1);double(1);double(1);double(1);double(1);double(1);double(1);double(1);double(1);double(1);double(1);double(1);double(1);double(1)]')  Offsets=str2num('[double(0);double(0);double(0);double(0);double(0);double(0);double(0);double(0);double(0);double(0);double(0);double(0);double(0);double(0)]')  Minimums=str2num('[double(0);double(0);double(0);double(0);double(0);double(0);double(-Inf);double(-Inf);double(0);double(0);double(0);double(0);double(0);double(0)]')  Maximums=str2num('[double(15);double(255);double(1);double(1);double(1);double(1);double(Inf);double(Inf);double(7);double(1);double(1);double(1);double(1);double(1)]')
      settings: DataFormat=CANdb specified signals
  CAN Unpack5 : canmsglib/CAN Unpack  CANdbFile=C:\Users\EcoCAR_HIL\Documents\Khanna\EcoSIM3_P1_0_PHEV_TCU\Final_DBC\20160113 RMS PM CAN DB.dbc  MsgList=M161_Temperature_Set_2  MsgName=M161_Temperature_Set_2  MsgIDType=Standard (11-bit identifier)  MsgIdentifier=161  MsgLength=8  SignalInfo=D1_Control_Board_Temperature$0$16$1$1$1$0$1.000000e-01$0$-3.276800e+03$3.276700e+03$#D2_RTD1_Temperature$16$16$1$1$1$0$1.000000e-01$0$-3.276800e+03$3.276700e+03$#D3_RTD2_Temperature$32$16$1$1$1$0$1.000000e-01$0$-3.276800e+03$3.276700e+03$#D4_RTD3_Temperature$48$16$1$1$1$0$1.000000e-01$0$-3.276800e+03$3.276700e+03$#  NSignals=4  IDPort=off  TimestampPort=off  ErrorPort=off  RemotePort=off  LengthPort=off  StatusPort=off  StartBits=str2num('[int32(0);int32(16);int32(32);int32(48)]')  SignalSizes=str2num('[int32(16);int32(16);int32(16);int32(16)]')  ByteOrders=str2num('[int32(1);int32(1);int32(1);int32(1)]')  DataTypes=str2num('[int32(1);int32(1);int32(1);int32(1)]')  MultiplexTypes=str2num('[int32(1);int32(1);int32(1);int32(1)]')  MultiplexValues=str2num('[double(0);double(0);double(0);double(0)]')  Factors=str2num('[double(1.000000e-01);double(1.000000e-01);double(1.000000e-01);double(1.000000e-01)]')  Offsets=str2num('[double(0);double(0);double(0);double(0)]')  Minimums=str2num('[double(-3.276800e+03);double(-3.276800e+03);double(-3.276800e+03);double(-3.276800e+03)]')  Maximums=str2num('[double(3.276700e+03);double(3.276700e+03);double(3.276700e+03);double(3.276700e+03)]')
      settings: DataFormat=CANdb specified signals
  CAN Unpack6 : canmsglib/CAN Unpack  CANdbFile=C:\Users\EcoCAR_HIL\Documents\Khanna\EcoSIM3_P1_0_PHEV_TCU\Final_DBC\20160113 RMS PM CAN DB.dbc  MsgList=M162_Temperature_Set_3  MsgName=M162_Temperature_Set_3  MsgIDType=Standard (11-bit identifier)  MsgIdentifier=162  MsgLength=8  SignalInfo=D1_RTD4_Temperature$0$16$1$1$1$0$1.000000e-01$0$-3.276800e+03$3.276700e+03$#D2_RTD5_Temperature$16$16$1$1$1$0$1.000000e-01$0$-3.276800e+03$3.276700e+03$#D3_Motor_Temperature$32$16$1$1$1$0$1.000000e-01$0$-3.276800e+03$3.276700e+03$#D4_Torque_Shudder$48$16$1$1$1$0$1.000000e-01$0$-3.276800e+03$3.276700e+03$#  NSignals=4  IDPort=off  TimestampPort=off  ErrorPort=off  RemotePort=off  LengthPort=off  StatusPort=off  StartBits=str2num('[int32(0);int32(16);int32(32);int32(48)]')  SignalSizes=str2num('[int32(16);int32(16);int32(16);int32(16)]')  ByteOrders=str2num('[int32(1);int32(1);int32(1);int32(1)]')  DataTypes=str2num('[int32(1);int32(1);int32(1);int32(1)]')  MultiplexTypes=str2num('[int32(1);int32(1);int32(1);int32(1)]')  MultiplexValues=str2num('[double(0);double(0);double(0);double(0)]')  Factors=str2num('[double(1.000000e-01);double(1.000000e-01);double(1.000000e-01);double(1.000000e-01)]')  Offsets=str2num('[double(0);double(0);double(0);double(0)]')  Minimums=str2num('[double(-3.276800e+03);double(-3.276800e+03);double(-3.276800e+03);double(-3.276800e+03)]')  Maximums=str2num('[double(3.276700e+03);double(3.276700e+03);double(3.276700e+03);double(3.276700e+03)]')
      settings: DataFormat=CANdb specified signals
  CAN Unpack8 : canmsglib/CAN Unpack  CANdbFile=C:\Users\EcoCAR_HIL\Documents\Khanna\EcoSIM3_P1_0_PHEV_TCU\Final_DBC\20160113 RMS PM CAN DB.dbc  MsgList=M172_Torque_And_Timer_Info  MsgName=M172_Torque_And_Timer_Info  MsgIDType=Standard (11-bit identifier)  MsgIdentifier=172  MsgLength=8  SignalInfo=D1_Commanded_Torque$0$16$1$1$1$0$1.000000e-01$0$-3.276800e+03$3.276700e+03$#D2_Torque_Feedback$16$16$1$1$1$0$1.000000e-01$0$-3.276800e+03$3.276700e+03$#D3_Power_On_Timer$32$32$1$2$1$0$3.000000e-03$0$0$4294970000$#  NSignals=3  IDPort=off  TimestampPort=off  ErrorPort=off  RemotePort=off  LengthPort=off  StatusPort=off  StartBits=str2num('[int32(0);int32(16);int32(32)]')  SignalSizes=str2num('[int32(16);int32(16);int32(32)]')  ByteOrders=str2num('[int32(1);int32(1);int32(1)]')  DataTypes=str2num('[int32(1);int32(1);int32(2)]')  MultiplexTypes=str2num('[int32(1);int32(1);int32(1)]')  MultiplexValues=str2num('[double(0);double(0);double(0)]')  Factors=str2num('[double(1.000000e-01);double(1.000000e-01);double(3.000000e-03)]')  Offsets=str2num('[double(0);double(0);double(0)]')  Minimums=str2num('[double(-3.276800e+03);double(-3.276800e+03);double(0)]')  Maximums=str2num('[double(3.276700e+03);double(3.276700e+03);double(4294970000)]')
      settings: DataFormat=CANdb specified signals
  Terminator{1,11,15..25,40} (14 alike) : Terminator
  Terminator_{22..32} (11 alike) : Terminator
  EMTransmit : Outport
  wires:
  Bus Creator4/1 -> Bus Creator8/3  "M170_Internal_States"
  CAN Unpack4/1 -> Bus Creator4/1  "VSM_State"
  CAN Unpack4/2 -> Terminator15/1
  CAN Unpack4/3 -> Terminator16/1
  CAN Unpack4/4 -> Terminator17/1
  CAN Unpack4/5 -> Terminator18/1
  CAN Unpack4/6 -> Terminator19/1
  CAN Unpack4/7 -> Terminator20/1
  CAN Unpack4/8 -> Terminator21/1
  CAN Unpack4/9 -> Terminator22/1
  CAN Unpack4/10 -> Terminator23/1
  CAN Unpack4/11 -> Terminator24/1
  CAN Unpack4/13 -> Terminator25/1
  CAN Unpack4/14 -> Bus Creator4/3  "Direction_Command_Feedback"
  CAN Unpack8/1 -> Terminator11/1
  CAN Unpack8/3 -> Terminator40/1
  CAN Unpack4/12 -> Bus Creator4/2  "Inverter_Enable_Lockout"
  CAN Unpack8/2 -> Bus Creator1/1  "EM_Torque_Out_Nm"
  CAN Receive1/1 -> Terminator1/1
  CAN Unpack1/2 -> Bus Creator2/1  "Motor_Speed"
  CAN Receive1/2 -> CAN Unpack3/1, CAN Unpack5/1, CAN Unpack6/1, CAN Unpack8/1, CAN Unpack4/1, CAN Unpack2/1, CAN Unpack1/1
  CAN Unpack2/1 -> Bus Creator3/1  "POST_Fault"
  CAN Unpack2/3 -> Bus Creator3/2  "RUN_Fault"
  CAN Unpack3/1 -> Bus Creator5/1  "Module_A"
  CAN Unpack3/2 -> Bus Creator5/2  "Module_B"
  CAN Unpack3/3 -> Bus Creator5/3  "Module_C"
  CAN Unpack3/4 -> Bus Creator5/4  "Gate_Driver_Board"
  CAN Unpack5/1 -> Bus Creator6/1  "Control_Board_Temperature"
  CAN Unpack6/3 -> Bus Creator7/1  "Motor_Temperature"
  Bus Creator3/1 -> Bus Creator8/1  "M171_Fault_Codes"
  Bus Creator2/1 -> Bus Creator8/2  "M165_Motor_Position_Info"
  Bus Creator1/1 -> Bus Creator8/4  "M172_Torque_And_Timer_Info"
  Bus Creator5/1 -> Bus Creator8/5  "M160_Temperature_Set_1"
  Bus Creator6/1 -> Bus Creator8/6  "M161_Temperature_Set_2"
  Bus Creator7/1 -> Bus Creator8/7  "M162_Temperature_Set_3"
  Bus Creator8/1 -> EMTransmit/1  "EM_CAN_Out"
  CAN Unpack1/1 -> Terminator_22/1
  CAN Unpack1/3 -> Terminator_23/1
  CAN Unpack1/4 -> Terminator_24/1
  CAN Unpack2/2 -> Terminator_25/1
  CAN Unpack2/4 -> Terminator_26/1
  CAN Unpack5/2 -> Terminator_27/1
  CAN Unpack5/3 -> Terminator_28/1
  CAN Unpack5/4 -> Terminator_29/1
  CAN Unpack6/1 -> Terminator_30/1
  CAN Unpack6/2 -> Terminator_31/1
  CAN Unpack6/4 -> Terminator_32/1

== system EcoSIM3_P2_C2_WIP/Supervisory Controller/Supervisory_IO/VNT Vector/CAN Rx/Engine ==
  Bus Creator : BusCreator  Inputs=1
  Bus Creator4 : BusCreator  Inputs=1
  CAN Receive1 : canlib/CAN Receive  BlockHandle=18086.0005  DeviceMenu=Vector Virtual 1 (Channel 1)  Device=Vector Virtual 1 (Channel 1)  ObjConstructor=canChannel('Vector', 'Virtual 1', 1)  EnableStandardIDsFilter=off  StandardIDs=104  EnableExtendedIDsFilter=off  ExtendedIDs=0  SampleTime=0.01  MsgsPerTimestep=1  StdIDsCombo=Allow only  ExtIDsCombo=Block all  InternalFilterUpdateStatus=on
  CAN Unpack1 : canmsglib/CAN Unpack  CANdbFile=C:\Users\EcoCAR_HIL\Documents\Khanna\EcoSIM3_P1_0_PHEV_TCU\Final_DBC\Engine_Transmission_BAS.dbc  MsgList=ECO_Engine_MSG104  MsgName=ECO_Engine_MSG104  MsgIDType=Standard (11-bit identifier)  MsgIdentifier=104  MsgLength=2  SignalInfo=ICE_Torque_Cmd_Nm$9$15$2$2$1$0$1.000000e-02$0$0$3.276700e+02$#  NSignals=1  IDPort=off  TimestampPort=off  ErrorPort=off  RemotePort=off  LengthPort=off  StatusPort=off  StartBits=str2num('[int32(9)]')  SignalSizes=str2num('[int32(15)]')  ByteOrders=str2num('[int32(2)]')  DataTypes=str2num('[int32(2)]')  MultiplexTypes=str2num('[int32(1)]')  MultiplexValues=str2num('[double(0)]')  Factors=str2num('[double(1.000000e-02)]')  Offsets=str2num('[double(0)]')  Minimums=str2num('[double(0)]')  Maximums=str2num('[double(3.276700e+02)]')
      settings: DataFormat=CANdb specified signals
  Terminator1 : Terminator
  ICETransmit : Outport
  wires:
  CAN Receive1/2 -> CAN Unpack1/1
  CAN Receive1/1 -> Terminator1/1
  CAN Unpack1/1 -> Bus Creator/1  "ICE_Torque_Cmd_Nm"
  Bus Creator/1 -> Bus Creator4/1  "ICE_Torque"
  Bus Creator4/1 -> ICETransmit/1  "ICE_CAN_Out"
